simulink model "robust_ES"  (R2024a)
settings: Solver=FixedStepAuto  StartTime=0.0  StopTime=300  FixedStep=0.0001  RelTol=1e-3
values from neighbouring files (symbols this model uses):
  a = 0.05    [prescribed_time_parameters.m]    (also in unbiased_ES_parameters.m)
  k = 0.01    [prescribed_time_parameters.m]    (also in unbiased_ES_parameters.m)
  lambda = 0.2    [prescribed_time_parameters.m]    (also in unbiased_ES_parameters.m = 0)
  w = 15    [prescribed_time_parameters.m]    (also in unbiased_ES_parameters.m = 5)
  wh = 3    [prescribed_time_parameters.m]    (also in unbiased_ES_parameters.m)
  wl = 3    [prescribed_time_parameters.m]    (also in unbiased_ES_parameters.m)
undefined symbols (not defined in the file or in its folder): National_Instruments, PCI
libraries: cstblocks x3, sldrtlib x2
settings Model: SimulationMode=external  ExtModeTrigDuration=3000001  ExtModeArchiveMode=auto  ExtModeArchiveFileName=seeking-data  ExtModeArchiveDirName=C:\Users\Eric\nonlinear-adaptive-control-lab-extremum-seeking-photovoltaic-experiment\tugrul-scripts\stored-data\robust-testing\robust-es  Creator=CTY  LastModifiedBy=Eric
settings HardwareCC: ProdBitPerLong=64  ProdHWDeviceType=Intel->x86-64 (Linux 64)
settings ModelReferenceCC: EnableRefExpFcnMdlSchedulingChecks=on
settings RTWCC: Description=Simulink Desktop Real-Time  SystemTargetFile=sldrt.tlc  TemplateMakefile=sldrt.tmf  TargetLang=C++  RTWCompilerOptimization=on  GPUComputeCapability=3.5
settings CodeAppCC: MaxIdLength=95
settings SimulinkDesktopRealTimeCC: TargetLibSuffix=_sldrt.a  TargetPreCompLibLocation=C:\Program Files\MATLAB\R2024a\toolbox\sldrt\lib\win64  TargetLangStandard=C++11 (ISO)

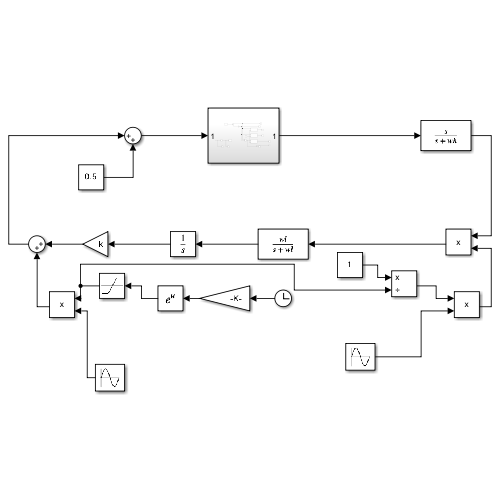
[thumbnail: Simulink's stored preview of the top-level diagram]
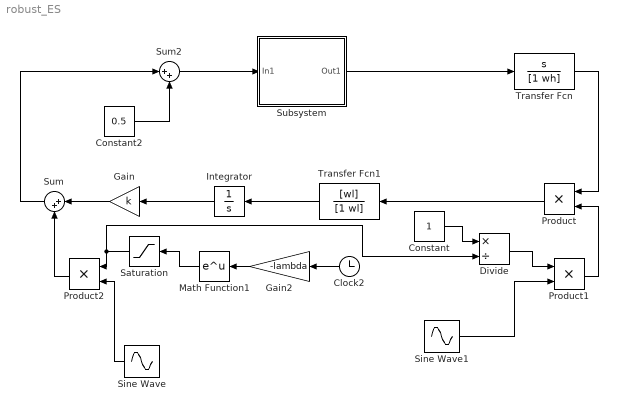
== system robust_ES ==
  Clock2 : Clock
  Constant : Constant
  Constant2 : Constant  Value=0.5
  Divide : Product  Inputs=*/
  Gain : Gain  Gain=k
  Gain2 : Gain  Gain=-lambda
  Integrator : Integrator
  Math Function1 : Math
  Product : Product
  Product1 : Product
  Product2 : Product
  Saturation : Saturate  UpperLimit=1.0  LowerLimit=0.2
  Sine Wave : Sin  Amplitude=a  Frequency=w  SampleTime=0
  Sine Wave1 : Sin  Amplitude=2/a  Frequency=w  SampleTime=0
  Subsystem : Subsystem
  Sum : Sum  Inputs=|++
  Sum2 : Sum  Inputs=|++
  Transfer Fcn : TransferFcn  Numerator=[1 0]  Denominator=[1 wh]
  Transfer Fcn1 : TransferFcn  Numerator=[wl]  Denominator=[1 wl]
  wires:
  Subsystem/1(Out1) -> Transfer Fcn/1
  Product/1 -> Transfer Fcn1/1
  Transfer Fcn/1 -> Product/1
  Product1/1 -> Product/2
  Transfer Fcn1/1 -> Integrator/1
  Product2/1 -> Sum/2
  Integrator/1 -> Gain/1
  Gain/1 -> Sum/1
  Sine Wave/1 -> Product2/2
  Sine Wave1/1 -> Product1/2
  Gain2/1 -> Math Function1/1
  Clock2/1 -> Gain2/1
  Constant/1 -> Divide/1
  Divide/1 -> Product1/1
  Math Function1/1 -> Saturation/1
  Sum/1 -> Sum2/1
  Sum2/1 -> Subsystem/1(In1)
  Constant2/1 -> Sum2/2
  Saturation/1 -> Divide/2, Product2/1

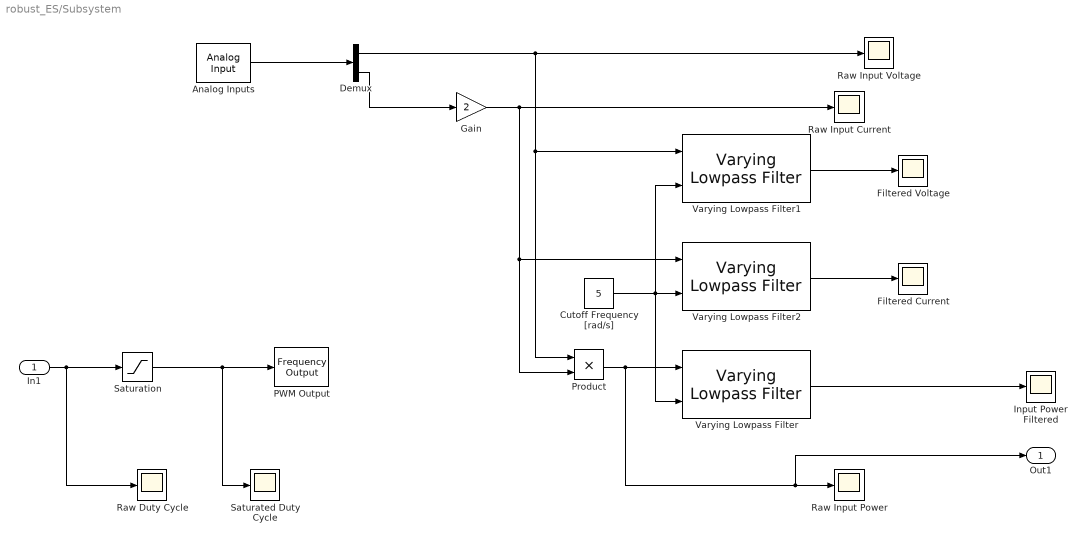
== system robust_ES/Subsystem ==
  In1 : Inport
  Analog Inputs : sldrtlib/Analog Input  SampleTime=0.001  MaxMissedTicks=100  ShowMissedTicks=off  YieldWhenWaiting=off  DrvName=National_Instruments/PCI-6251  DrvAddress=4294967295  DrvOptions=[1 0 0 3 3]  Channels=[1, 2]  RangeMode=1  VoltRange=1  DataType=1
      settings: AttributesFormatString=National Instruments\nPCI-6251 [auto]
  Cutoff Frequency [rad/s] : Constant  Value=5
  Demux : Demux  Outputs=2
  Filtered Current : Scope
  Filtered Voltage : Scope
  Gain : Gain  Gain=2
  Input Power Filtered : Scope
  PWM Output : sldrtlib/Frequency Output  SampleTime=0.0001  MaxMissedTicks=100000  ShowMissedTicks=off  YieldWhenWaiting=off  DrvName=National_Instruments/PCI-6251  DrvAddress=4294967295  DrvOptions=[1 0 0 3 3]  Channels=1  FrequencySource=1  Frequency=200000  FrequencyFinalValue=[]  DutySource=2  Duty=[]  DutyFinalValue=[]
      settings: AttributesFormatString=National Instruments\nPCI-6251 [auto]
  Product : Product
  Raw Duty Cycle : Scope
  Raw Input Current : Scope
  Raw Input Power : Scope
  Raw Input Voltage : Scope
  Saturated Duty Cycle : Scope
  Saturation : Saturate  UpperLimit=0.9  LowerLimit=0.2
  Varying Lowpass Filter : cstblocks/Linear Parameter Varying/Varying Lowpass Filter  N=1
  Varying Lowpass Filter1 : cstblocks/Linear Parameter Varying/Varying Lowpass Filter  N=1
  Varying Lowpass Filter2 : cstblocks/Linear Parameter Varying/Varying Lowpass Filter  N=1
  Out1 : Outport
  wires:
  Saturation/1 -> Saturated Duty Cycle/1, PWM Output/1
  Varying Lowpass Filter/1 -> Input Power Filtered/1
  Gain/1 -> Raw Input Current/1, Varying Lowpass Filter2/1, Product/2
  Varying Lowpass Filter1/1 -> Filtered Voltage/1
  Cutoff Frequency [rad/s]/1 -> Varying Lowpass Filter1/2, Varying Lowpass Filter2/2, Varying Lowpass Filter/2
  Demux/1 -> Raw Input Voltage/1, Varying Lowpass Filter1/1, Product/1
  In1/1 -> Raw Duty Cycle/1, Saturation/1
  Varying Lowpass Filter2/1 -> Filtered Current/1
  Analog Inputs/1 -> Demux/1
  Product/1 -> Out1/1, Raw Input Power/1, Varying Lowpass Filter/1
  Demux/2 -> Gain/1
